simulink model "LongLatDriveline"  (R2024b)
settings: Solver=FixedStepAuto  StartTime=0  StopTime=120  FixedStep=0.002  RelTol=1e-3
InitFcn:
  | load('waypoints.mat');
  | VehicleObj = Simulink.data.dictionary.open('./ModelData/VehicleData.sldd');
  | %dDataSectObj = getSection(myDictionaryObj,'Design Data');
StopFcn:
  | Plot_LateralModelErrorControl;
  | 
  | mdlWks = get_param(gcs, 'ModelWorkspace');
  | par_ToDrvDesigner = evalin(mdlWks, 'ToDrvDesigner');
  | 
  | if par_ToDrvDesigner.Value
  |     ExportdrivingScenario;
  | end
model workspace (MAT data in the model file):
  ToDrvDesigner : Simulink.Parameter (value not decoded)
values from neighbouring files (symbols this model uses):
  A_F = 2.341157    [VehicleData.sldd]
  C_af = 80000.0    [VehicleData.sldd]
  C_ar = 80000.0    [VehicleData.sldd]
  C_d = 0.24    [VehicleData.sldd]
  f = 0.01    [VehicleData.sldd]
  g = 9.81    [VehicleData.sldd]
  h_aero = 0.65    [VehicleData.sldd]
  h_gc = 0.65    [VehicleData.sldd]
  Iz = 2873.0    [VehicleData.sldd]
  lf = 1.1    [VehicleData.sldd]
  lr = 1.58    [VehicleData.sldd]
  m = 2238.932    [VehicleData.sldd]
  Nf = 2.0    [VehicleData.sldd]
  Nr = 2.0    [VehicleData.sldd]
  r_stat = 0.342    [VehicleData.sldd]
  r_w = 0.352    [VehicleData.sldd]
  rho = 1.225    [VehicleData.sldd]
  theta = 0.0    [VehicleData.sldd]
  transGear = 0.1027    [VehicleData.sldd]
  V_wind = 0.0    [VehicleData.sldd]
symbols that are objects in the model workspace (value not decoded): ToDrvDesigner
undefined symbols (not defined in the file or in its folder): InitialPsi, InitialX, InitialY, phi
libraries: slpidlib x14, spsMosfetLib x6, simulink x4, spsVoltageMeasurementLib x3, SignalEditorBlockLib x2, spsDCVoltageSourceLib x1, spspowerguiLib x1
(part 3 of 5)

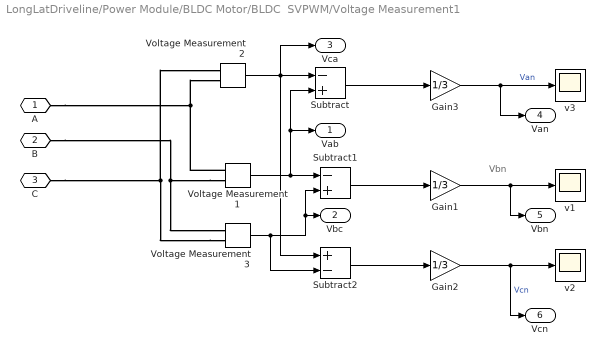
== system LongLatDriveline/Power Module/BLDC Motor/BLDC  SVPWM/Voltage Measurement1 ==
  note: Vbn
  Gain1 : Gain  Gain=1/3
  Gain2 : Gain  Gain=1/3
  Gain3 : Gain  Gain=1/3
  Subtract : Sum  Inputs=-+
  Subtract1 : Sum  Inputs=-+
  Subtract2 : Sum  Inputs=+-
  Voltage Measurement1 : spsVoltageMeasurementLib/Voltage Measurement  PhasorSimulation=off  OutputType=Complex  PSBequivalent=0
  Voltage Measurement2 : spsVoltageMeasurementLib/Voltage Measurement  PhasorSimulation=off  OutputType=Complex  PSBequivalent=0
  Voltage Measurement3 : spsVoltageMeasurementLib/Voltage Measurement  PhasorSimulation=off  OutputType=Complex  PSBequivalent=0
  v1 : Scope
  v2 : Scope
  v3 : Scope
  A : PMIOPort  Side=Left
  B : PMIOPort  Port=2  Side=Left
  C : PMIOPort  Port=3  Side=Left
  Vab : Outport  VectorParamsAs1DForOutWhenUnconnected=off
  Vbc : Outport  Port=2  VectorParamsAs1DForOutWhenUnconnected=off
  Vca : Outport  Port=3  VectorParamsAs1DForOutWhenUnconnected=off
  Van : Outport  Port=4  VectorParamsAs1DForOutWhenUnconnected=off
  Vbn : Outport  Port=5  VectorParamsAs1DForOutWhenUnconnected=off
  Vcn : Outport  Port=6  VectorParamsAs1DForOutWhenUnconnected=off
  wires:
  Gain2/1 -> v2/1, Vcn/1  "Vcn"
  Subtract2/1 -> Gain2/1
  Gain1/1 -> v1/1, Vbn/1
  Subtract1/1 -> Gain1/1
  Voltage Measurement3/1 -> Subtract1/2, Vbc/1, Subtract2/2
  Gain3/1 -> v3/1, Van/1  "Van"
  Subtract/1 -> Gain3/1
  Voltage Measurement1/1 -> Vab/1, Subtract/2, Subtract1/1
  Voltage Measurement2/1 -> Vca/1, Subtract2/1, Subtract/1
  connections:
  Voltage Measurement1/LConn1 -- A/RConn1 -- Voltage Measurement2/LConn2
  Voltage Measurement1/LConn2 -- B/RConn1 -- Voltage Measurement3/LConn1
  Voltage Measurement3/LConn2 -- Voltage Measurement2/LConn1 -- C/RConn1

== system LongLatDriveline/Vehicle Lateral Model/DynamicModel/LateralDynamics/LateralDynamicWithNoise ==
  note: This variant does not simplify the small angle tan. i.e. tan(x) = x
  X : Inport
  Vx : Inport  Port=2
  dd : Inport  Port=3
  phi_ref : Inport  Port=4
  LateralDynamicWithNoise : MATLAB Function  TreatAsAtomicUnit=on  VariantControl=NotSimplifiedModel
  Sine Wave : Sin  Amplitude=0.6  Frequency=(2*pi)/8  SampleTime=0
  Sine Wave1 : Sin  Amplitude=pi/60  Frequency=pi/8  SampleTime=0
  dX : Outport
  wires:
  X/1 -> LateralDynamicWithNoise/1(X)
  Vx/1 -> LateralDynamicWithNoise/2(Vx)
  dd/1 -> LateralDynamicWithNoise/3(dd)
  LateralDynamicWithNoise/1(dX) -> dX/1
  phi_ref/1 -> LateralDynamicWithNoise/4(phi_ref)
  Sine Wave/1 -> LateralDynamicWithNoise/5(NoiseDdy)
  Sine Wave1/1 -> LateralDynamicWithNoise/6(NoiseDdpsi)

== system LongLatDriveline/Power Module/BLDC Motor/BLDC  SVPWM/SVPWM Generator/Timer ==
  note: It triggers the output when the time is greatter or equal to the input in seconds
  time : Inport
  Add2 : Sum
  Constant13 : Constant
  Constant14 : Constant  Value=0
  Relational Operator : RelationalOperator  OutDataTypeStr=boolean  RndMeth=Simplest  InputSameDT=off
  Switch : Switch  Criteria=u2 > Threshold  SaturateOnIntegerOverflow=off  InputSameDT=off
  Unit Delay : UnitDelay  SampleTime=-1  HasFrameUpgradeWarning=on
  Weighted Sample Time : SampleTimeMath  TsampMathOp=Ts Only
  trigger : Outport
  wires:
  Switch/1 -> Unit Delay/1
  Add2/1 -> Relational Operator/1, Switch/3
  Relational Operator/1 -> trigger/1, Switch/2
  Weighted Sample Time/1 -> Add2/1
  Constant13/1 -> Weighted Sample Time/1
  Constant14/1 -> Switch/1
  Unit Delay/1 -> Add2/2
  time/1 -> Relational Operator/2

== system LongLatDriveline/Power Module/BLDC Motor/BLDC  SVPWM/SVPWM Generator/count14 ==
  Trigger : TriggerPort  VariantControl=(inherit)
  Add : Sum
  Compare To Constant : simulink/Logic and Bit Operations/Compare To Constant  relop=>=  const=4  OutDataTypeStr=boolean
  Compare To Constant1 : simulink/Logic and Bit Operations/Compare To Constant  relop=<=  const=1  OutDataTypeStr=boolean
  Constant : Constant  Value=-1
  Constant1 : Constant
  Switch : Switch  Criteria=u2 > Threshold  Threshold=1  SaturateOnIntegerOverflow=off  InputSameDT=off
  Switch1 : Switch  Criteria=u2 > Threshold  Threshold=1  SaturateOnIntegerOverflow=off  InputSameDT=off
  Unit Delay : UnitDelay  InitialCondition=1  SampleTime=-1  HasFrameUpgradeWarning=on
  Unit Delay1 : UnitDelay  InitialCondition=1  SampleTime=-1  HasFrameUpgradeWarning=on
  count : Outport  InitialOutput=1
  wires:
  Add/1 -> Unit Delay/1, count/1, Compare To Constant/1, Compare To Constant1/1
  Unit Delay/1 -> Add/2
  Unit Delay1/1 -> Switch/3, Add/1
  Constant/1 -> Switch/1
  Switch/1 -> Switch1/3
  Switch1/1 -> Unit Delay1/1
  Compare To Constant/1 -> Switch/2
  Compare To Constant1/1 -> Switch1/2
  Constant1/1 -> Switch1/1

== matlab function LongLatDriveline/Tyre ModelV1/TireSlip ==
  data: Vx input; s_xf output; w_wf input; r_eff input
%BASED ON
%Rajesh Rajamani, Vehicle Dynamics and Control, Minneapolis, MN, Springer, 2012.
%Chapter 4.1.2
function s_xf = XTireSlip(Vx,w_wf,r_eff) 

if Vx == 0
   s_xf = 0.1 * sign(w_wf);   
else
   s_xf = (r_eff*w_wf -Vx)/abs(Vx); % acceleration
end

if s_xf > 1
   %s_xf = 1; 
end

== matlab function LongLatDriveline/LateralController/SMC_Alcala/AlcalaSMC ==
  data: U output size=1; E input; Vx input; dPsi_des input; dx_e input; ddPsi_des input; C_af parameter; g parameter; C_ar parameter; lf parameter; lr parameter; Iz parameter; m parameter
% ******************* Lateral dynamic controller *********************
%*********************************************************************
% Author: L.Arturo Torres-Romero
% Date: 22-10-2020
% This controller controlls the direction of a car, based in the dynamics
% described  in the next link and using the Direct Lyapunov formulation: 
% https://www.researchgate.net/publication/340166902_LATERAL_VEHICLE_DYNAMICS_AND_CONTROLLERS_DESIGN
%
%ALCALÁ, Eugenio, et al. Comparison of two non-linear model-based control strategies for autonomous vehicles. 
% En 2016 24th Mediterranean Conference on Control and Automation (MED). IEEE, 2016. p. 846-851.
%******************* PARAMETERS DESCRIPTIONS **********************
%******************************************************************
% m: vehicle mass
% g: gravity
% C_af : Cornering  stiffness  of  front  wheels.
% C_ar : Cornering  stiffness  of  rear  wheels.
% lf : distance fron the center of gravity to the front wheel axis.
% lr : distance fron the center of gravity to the rear wheel axis.
% Iz : this is the momentum of inertia of the vehicle respect the z axis.
%******************************************************************
%******************* INPUTS DESCRIPTIONS **************************
%******************************************************************
% E:   (column vector)[e1;de1;e2;de2] states of the state space of 
%       the system that includes the errors as follows:
%      e1  : is the lateral position error respect the road.
%      de1 : derivative of e1.
%      e2  : is the yaw angle error with respect the road. 
%      de2 : derivarive of the e2.
% Vx: Logitudinal velocity.

%******************************************************************
% ******************* OUTPUTS DESCRIPTIONS ************************
%******************************************************************
% U: control coutput in radians. Angle of the frontal wheels respect to the
%    longitudinal axis
% isCtrl: when true means that the matrix Mc has full rank, and hence, the
%         system is controllable
%******************************************************************

function U = SMC_Ctrl_1(E, Vx,dPsi_des,dx_e,ddPsi_des, C_af, g, C_ar, lf, lr, Iz, m) % pd polos deseados
y_e = E(1);
dy_e = E(2);
psi_e = E(3);
dpsi_e = E(4);
x_e = E(5);


L = lf+lr;
k2 = 2;
k3 = 2.55;
P2 = 3.7;
Q2 = 0.3;

s2 = dy_e +k2*y_e + k3*psi_e;

dPsi_ctrl = dPsi_des + (-P2*s2 -Q2*sign(s2) -k2*dy_e + ddPsi_des*x_e + dPsi_des*dx_e  -Vx*sin(psi_e))/(Vx*sin(psi_e)+k3);

ctrlVal = atan((L*dPsi_ctrl)/Vx);

U = real(ctrlVal);

== matlab function LongLatDriveline/Tyre ModelV1/WheelsDynamic ==
  data: T_wheels input; dw_wf output; r_eff output; F_xf input; r_w parameter; r_stat parameter
% ******************* Wheel inertia dynamics *********************
%****************************************************************
% BASED ON 
% Rajesh Rajamani, Vehicle Dynamics and Control, Minneapolis, MN, Springer, 2012.
%Chapter 4.2.4
% r_eff = effective radius of the wheel
% F_xf = longitudinal tire force from the front wheels
function [dw_wf, r_eff]= fcn(T_wheels,F_xf, r_w, r_stat)

%r_w = 0.352; % radius of the tire. Pirelli Sottozero 3 P245/45WR19
%r_stat = 0.342; % static vertical deflection of the tire
alpha = acos(r_stat/r_w);
r_eff = (alpha*r_w)/alpha;

I_w = .9; % TODO define this
dw_wf = (T_wheels -(r_eff*F_xf))/I_w;

== matlab function LongLatDriveline/Power Module/BLDC Motor/BLDC  SVPWM/InvPark ==
  data: X_dq input size=[2 1]; Y_ab0 output; theta input
function Y_ab0 = fcn(X_dq, theta)
X_dq0 = [X_dq; 0];

%inverse Park 
iT_C = [cos(theta)   -sin(theta)    0; ...
        sin(theta)    cos(theta)    0; ...
        0             0             1];
%               
             
Y_ab0 =iT_C*X_dq0;
end

== matlab function LongLatDriveline/Tyre ModelV2/MagicFormula ==
  data: X input; Y output; F_zf input
%BASED ON
%Massimo Guiggiani, The Science of Vehicle Dynamics, Pisa, Italy, Springer Netherlands, 2014.
%Chapter 2.12
%The values of the MF were obtained from the graph in fig. 2.22
function Y = XTireForce(X, F_zf) 
% B stiffness factor
% C shape factor
% D peak value
% E curvature factor
% Sh horizontal shift
% Sv vertical shift

Sh = 0;% Sh horizontal shift
Sv = 0; %vertical shift

D = 3; % ym, maximum value Experimental from graph
C = 1.5;
B = 20;
E = 0;

x = X-Sh;
gamma = C*atan(B*x-E*(B*x-atan(B*x)));
y = F_zf*D*sin(gamma);
Y = (y - Sv);

== matlab function LongLatDriveline/Tyre ModelV2/TireSlip ==
  data: Vx input; s_xf output; w_wf input; r_eff input
%BASED ON
%Rajesh Rajamani, Vehicle Dynamics and Control, Minneapolis, MN, Springer, 2012.
%Chapter 4.1.2
function s_xf = XTireSlip(Vx,w_wf,r_eff) 

if Vx == 0
   s_xf = 0.1 * sign(w_wf);   
else
   s_xf = (r_eff*w_wf -Vx)/abs(Vx); % acceleration
end

if s_xf > 1
   %s_xf = 1; 
end

== matlab function LongLatDriveline/Power Module/SIEngineModel/SI_Engine/FrictionLosses ==
  data: w_e input; T_f output; p_man input
function T_f = fcn(w_e, p_man)
% According Heywood 98 friction loss = .97 +0.15*(N/1000)+  0.05(N/1000)^2
% Where N is RPM. here it is converted to rad/s



a0 = 4.559432e-6;
a1 = 0.009550;
a2 = .97;
b0 = 0;
b1 = 0;




T_f = abs(a0*w_e^2 + a1*w_e + a2 + b0*w_e*p_man + b1*p_man);a1*w_e + a2 + b0*w_e*p_man + b1*p_man;

== matlab function LongLatDriveline/Power Module/BLDC Motor/BLDC  SVPWM/MATLAB Function ==
  data: r output; x input; theta output; y input
function [r, theta] = rec2polar(x, y)

r = sqrt(x^2 + y^2);
theta = atan2(y,x);

== matlab function LongLatDriveline/Power Module/DC Motor/DC Motor ==
  data: X input; dX output; u input size=3; T output
function [dX, T]= fcn(X,u)
ia = X(1);
Va = u(1); wm =u(2); dwm =u(3);

MaxT = 800;

Ra = 0.193;
La = 0.00383;
Jm = 0.6;
Bm = 2.632177;
Kb = 2.332232;
KT = 2.1717;

A1 = -Ra/La;
B1 = [1/La -Kb/La 0];
C1 = KT;
D1 = [0 -Bm -Jm];

dX = A1*X + B1*u;
T = C1*X + D1*u;

if T > MaxT
    T = MaxT;
end
if T < 0
    T = 0;
end

end

== matlab function LongLatDriveline/Power Module/SIEngineModel/SI_Engine/InflowRateManifold ==
  data: alpha input; dm_ai output; p_man input
function dm_ai = fcn(alpha,p_man)

% Max  Automotive Powertrain Modeling for Control (D.Cho and J. K. Hedrick)
MAX = 0.1843; % Kg/s constant dependent on the size of the throttle body and is equalto the maximum possible intake airflow rate.
alpha_p = 0.05; %the minimum throttle angle seen by the engine.
pc = 0.5283; % critical pressure ratio
p_amb =101325; % pressure of 1 atm in Pa
p_r = p_man/p_amb;

if p_r <= pc
PRI = 1; % p_r <= pc Sonic
else
PRI = sqrt(1-((p_r-pc)/(1-pc))^2); % P_r > pc   chocked
end

TC = 1-cos(alpha-alpha_p);
dm_ai = MAX * TC * PRI;

== matlab function LongLatDriveline/Power Module/SIEngineModel/SI_Engine/ManifoldPressure ==
  data: dm_ao input; dm_ai input; dp_man output
function dp_man = fcn(dm_ao,dm_ai)
R = 8.314472; % (J/(K*mol)) ideal gas constant.
T_man = 60; % intake manifold temperature.
V_man = 1; % intake manifold volume

dp_man = (R*T_man*(dm_ai-dm_ao))/V_man;

== matlab function LongLatDriveline/LongitudinalDynamics ==
  data: F_xf input; dVx output; F_xr input; Vx input; rho parameter; g parameter; A_F parameter; C_d parameter; f parameter; m parameter; V_wind parameter; theta parameter; F_zf output; F_zr output; h_aero parameter; h_gc parameter; lf parameter; lr parameter; Nf parameter; Nr parameter
% BASED ON
% Rajesh Rajamani, Vehicle Dynamics and Control, Minneapolis, MN, Springer, 2012.
%Chapter 4.1

function [dVx,F_zf, F_zr] = LongitudinalDynamics(F_xf,F_xr,Vx, rho, g, A_F, C_d, f, m, V_wind, theta, h_aero, h_gc, lf, lr, Nf, Nr)
% m = 2238.932; % TESLA model S P85D
% g = 9.81;
% theta = 0;
% A_F = 2.341157; % Fontal area of the vehicle. TESLA model S P85D
% C_d  =0.24; %Ford Focus Aerodynamic drag coeficient. TESLA model S P85D
% rho = 1.225;  %(kg/m^3) Air density
% f = 0.01; % varies from 0.01 to 0.04
% V_wind = 0;
% Nf, Nr Number of wheels in front and rear axles

F_aero = (1/2)*rho*C_d*A_F*(Vx+V_wind)^2;

dVx = (F_xf + F_xr - F_aero - m*g*sin(theta))/m;

F_zf = (-F_aero*h_aero -m*dVx*h_gc -m*g*h_gc*sin(theta) +m*g*lr*cos(theta))/(Nf*(lr+lf));
F_zr = ( F_aero*h_aero +m*dVx*h_gc +m*g*h_gc*sin(theta) +m*g*lf*cos(theta))/(Nr*(lr+lf));

== matlab function LongLatDriveline/Power Module/SIEngineModel/SI_Engine/OutflowRateManifold ==
  data: w_e input; dm_ao output; p_man input; T_man input; ma input
function dm_ao = fcn(w_e, p_man, T_man,ma)
Vd = 0.0038; %displacement volume of the engine cylinders
R = 8.31446261815324; %constant used in ideal gas law for intake manifold

%volumetric efficiency

% Automotive Powertrain Modeling for Control (D.Cho and J. K. Hedrick)
eta_vol = (24.5*w_e -3.1e4)*ma^2 + (-1.167*w_e+222)*ma +(8.1e-4*w_e+0.352);
%eta_vol = 0.9;

dm_ao = ((eta_vol*w_e*Vd)/(4*pi))*(p_man/(R*T_man));

== matlab function LongLatDriveline/Power Module/SIEngineModel/SI_Engine/indTorque ==
  data: w_e input; T_ind output; dm_ao input
function T_ind = fcn(w_e, dm_ao)
% dm_ao: air mass flow rate out of the intake manifold and into the cylinder
% dm_f:  is the mass fuel rate into the cylinders 
H_u = 46000000; % fuel energy constant. look in other sources 44-46 MJ/kg found as (Gasoline heating value)
h_i = 0.45; % Thermal efficiency multiplier. Otto engine value.   from (Hendricks and Sorenson, 1990)
lambda = 1; % air/fuel equivalence ratio
L_th = 14.67; % stoichiometric air/fuel mass ratio for gasoline.


dm_f = dm_ao/(L_th*lambda);

if w_e ~= 0
T_ind = (H_u*h_i*dm_f)/w_e;   
else
T_ind = (H_u*h_i*dm_f)/0.01;    
end

== matlab function LongLatDriveline/Power Module/BLDC Motor/BLDC  SVPWM/Motor BLDC1 ==
  data: X input; dX output; Fabc input; u input; Wm input; dWm input; Tl output
function [dX, Tl] = fcn(X, Fabc, u, Wm, dWm)

== matlab function LongLatDriveline/Tyre ModelV2/WheelsDynamic ==
  data: T_wheels input; dw_wf output; r_eff output; F_xf input; r_w parameter; r_stat parameter
% ******************* Wheel inertia dynamics *********************
%****************************************************************
% BASED ON 
% Rajesh Rajamani, Vehicle Dynamics and Control, Minneapolis, MN, Springer, 2012.
%Chapter 4.2.4
% r_eff = effective radius of the wheel
% F_xf = longitudinal tire force from the front wheels
function [dw_wf, r_eff]= fcn(T_wheels,F_xf, r_w, r_stat)

%r_w = 0.352; % radius of the tire. Pirelli Sottozero 3 P245/45WR19
%r_stat = 0.342; % static vertical deflection of the tire
alpha = acos(r_stat/r_w);
r_eff = (alpha*r_w)/alpha;

I_w = .9; % TODO define this
dw_wf = (T_wheels -(r_eff*F_xf))/I_w;

== matlab function LongLatDriveline/Power Module/BLDC Motor/BLDC  SVPWM/ParkClarke4 ==
  data: X_abc input; Y_dq output; theta input
function Y_dq = fcn(X_abc, theta)

% Park clarke transform eliminating the third element
PC_T = (sqrt(2)/2)*[sqrt(3)*cos(theta)  sin(theta)  -sin(theta) ; ...
                    -sqrt(3)*sin(theta)  cos(theta)  -cos(theta)];

Y_dq =PC_T*X_abc;
end

== matlab function LongLatDriveline/Power Module/BLDC Motor/BLDC  SVPWM/SVPWM Generator/bin2vector ==
  data: y output; data input
function y = binary2vector(data)
y = [0; 0; 0];
g = dec2bin(data,3);
out = g-'0';
y(1) = out(1);
y(2) = out(2);
y(3) = out(3);


% powOf2 = 2.^[0:nBits-1];
% 
% %# do a tiny bit of error-checking
% if data > sum(powOf2)
%    error('not enough bits to represent the data')
% end
% 
% out = false(1,nBits);
% 
% ct = nBits;
% 
% while data>0
% if data >= powOf2(ct)
% data = data-powOf2(ct);
% out(ct) = true;
% end
% ct = ct - 1;
% end

== matlab function LongLatDriveline/Power Module/BLDC Motor/BLDC  SVPWM/Space Vector calculator ==
  data: n output; v output; theta_vs output; V_link input; Vs input; theta_vs1 input
function [n,v,theta_vs]= SpaceVectorCalc(V_link,Vs,theta_vs1)
v = [0 0];
theta_vs = mod(theta_vs1,2*pi);
theta = 0;
n = 0; % This is the quadrant of the vector. you should never get zero as output

if 0*(pi/180) <= theta_vs && theta_vs < 60*(pi/180)
   theta = theta_vs;
   n = 1;
elseif 60*(pi/180) <= theta_vs && theta_vs < 120*(pi/180)
   theta = theta_vs - 60*(pi/180);
   n = 2;
elseif 120*(pi/180) <= theta_vs && theta_vs < 180*(pi/180)  
    theta = theta_vs - 2*60*(pi/180);
    n = 3;
elseif 180*(pi/180) <= theta_vs && theta_vs < 240*(pi/180)  
    theta = theta_vs - 3*60*(pi/180);
    n = 4;
elseif 240*(pi/180) <= theta_vs && theta_vs < 300*(pi/180)
    theta = theta_vs - 4*60*(pi/180);
    n = 5;
elseif 300*(pi/180) <= theta_vs && theta_vs < 360*(pi/180)
    theta = theta_vs - 5*60*(pi/180);
    n = 6;
end


V_b = ((2*Vs)/sqrt(3))*sin(theta);
V_a = ((2*Vs)/sqrt(3))*sin(pi/3 - theta);

v = [V_a V_b];

== matlab function LongLatDriveline/Transmission ==
  data: T_wheels output; T_t input; w_t output; w_w input; R input
% ***************** Transmission ******************
% *************************************************
% BASED ON
% Rajesh Rajamani, Vehicle Dynamics and Control, Minneapolis, MN, Springer, 2012.
% Chapter 4.2.2
% T_wheels = wheels torque
% w_w = wheels angular speed
% R = gear ratio of transmission
%**************************************************

function [T_wheels, w_t]= fcn(T_t,w_w,R)

T_wheels = T_t/R;
w_t = w_w/R;
% itneed to be implemented "during change"

== matlab function LongLatDriveline/Power Module/BLDC Motor/BLDC abcModel/Fases abc ==
  data: X input; Fabc output
function Fabc = fcn(X)
    theta = mod(X(1),2*pi);
    
    if (0<=theta)&&(theta<(pi/6))
        Fa = (6/pi)*theta;
    elseif ((pi/6)<=theta)&&(theta<(5*pi/6))
        Fa = 1;
    elseif ((5*pi/6<=theta))&&(theta<(7*pi/6))
        Fa = (6/pi)*(pi-theta);
    elseif ((7*pi/6)<=theta)&&(theta<(11*pi/6))
        Fa = -1;
    elseif ((11*pi/6)<=theta)&&(theta<(2*pi))
        Fa = (6/pi)*(theta-2*pi);
    else
        Fa = NaN;
    end
    
    if (0<=theta)&&(theta<(3*pi/6))
        Fb = -1;
    elseif ((3*pi/6)<=theta)&&(theta<(5*pi/6))
        Fb = (6/pi)*(theta-(2*pi)/3);
    elseif ((5*pi/6)<=theta)&&(theta<(9*pi/6))
        Fb = 1;
    elseif ((9*pi/6)<=theta)&&(theta<(11*pi/6))
        Fb = (6/pi)*(-theta+(5*pi)/3);
    elseif ((11*pi/6)<=theta)&&(theta<(2*pi))
        Fb = -1;
    else
        Fb = NaN;
    end
    
    if (0<=theta)&&(theta<(pi/6))
        Fc = 1;
    elseif ((pi/6)<=theta)&&(theta<(3*pi/6))
        Fc = (6/pi)*(pi/3-theta);
    elseif ((3*pi/6)<=theta)&&(theta<(7*pi/6))
        Fc = -1;
    elseif ((7*pi/6)<=theta)&&(theta<(9*pi/6))
        Fc = (6/pi)*(theta-(4*pi)/3);
    elseif ((9*pi/6)<=theta)&&(theta<(2*pi))
        Fc = 1;
    else
        Fc = NaN; 
    end
    
    Fabc = [Fa;Fb;Fc];
end

== matlab function LongLatDriveline/Power Module/BLDC Motor/BLDC abcModel/Graphs ==
  data: X input; theta output; Iabc output
function [theta,Iabc] = DEMUX(X)
theta = X(1);Iabc = X(2:4);

== matlab function LongLatDriveline/Power Module/BLDC Motor/BLDC abcModel/Motor BLDC ==
  data: X input; dX output; Fabc input; u input; Wm input; dWm input; Tl output
function [dX,Tl] = fcn(X,Fabc,u,Wm,dWm)
Iabc = X(2:4);
R = 0.7;
L = 0.005;%0.00272-0.0015; %=L-Lm
J = 0.000284;
b = 0.02;
P = 4;
maxTl = 400; % max torque of the motor
Lambda = 0.105;

Vabc = u*Fabc;

Eabc = Lambda*Wm*Fabc;
dTheta = P*Wm/2;

if Wm > 0.01
Te = (Iabc'*Eabc)/Wm;
Tl = Te-b*Wm-J*dWm;
else
Tl  = maxTl;
end

if Tl > maxTl
Tl = maxTl;   
end

dIabc = (-R*Iabc - Eabc + Vabc)/L;

dX = [dTheta;dIabc];
end

== matlab function LongLatDriveline/Power Module/BLDC Motor/BLDC dqControl/Back EMF ==
  data: X input; Fabc output
function Fabc = fcn(X)
Fabc = [0;0;0];
    theta = mod(X(1),2*pi); %X(4)
    %theta = mod(X,2*pi);
    
    if (0<=theta)&&(theta<(pi/6))
        Fa = (6/pi)*theta;
    elseif ((pi/6)<=theta)&&(theta<(5*pi/6))
        Fa = 1;
    elseif ((5*pi/6<=theta))&&(theta<(7*pi/6))
        Fa = (6/pi)*(pi-theta);
    elseif ((7*pi/6)<=theta)&&(theta<(11*pi/6))
        Fa = -1;
    elseif ((11*pi/6)<=theta)&&(theta<(2*pi))
        Fa = (6/pi)*(theta-2*pi);
    else
        Fa = NaN;
    end
    
    if (0<=theta)&&(theta<(3*pi/6))
        Fb = -1;
    elseif ((3*pi/6)<=theta)&&(theta<(5*pi/6))
        Fb = (6/pi)*(theta-(2*pi)/3);
    elseif ((5*pi/6)<=theta)&&(theta<(9*pi/6))
        Fb = 1;
    elseif ((9*pi/6)<=theta)&&(theta<(11*pi/6))
        Fb = (6/pi)*(-theta+(5*pi)/3);
    elseif ((11*pi/6)<=theta)&&(theta<(2*pi))
        Fb = -1;
    else
        Fb = NaN;
    end
    
    if (0<=theta)&&(theta<(pi/6))
        Fc = 1;
    elseif ((pi/6)<=theta)&&(theta<(3*pi/6))
        Fc = (6/pi)*(pi/3-theta);
    elseif ((3*pi/6)<=theta)&&(theta<(7*pi/6))
        Fc = -1;
    elseif ((7*pi/6)<=theta)&&(theta<(9*pi/6))
        Fc = (6/pi)*(theta-(4*pi)/3);
    elseif ((9*pi/6)<=theta)&&(theta<(2*pi))
        Fc = 1;
    else
        Fc = NaN; 
    end
    
    
%     
     %Fa = sin(theta);
     %Fb = sin(theta - 2*pi/3);
     %Fc = sin(theta + 2*pi/3);
    
    Fabc = [Fa;Fb;Fc];
end

== matlab function LongLatDriveline/LateralController/SMC_UrbanoPathFollowing/SMC_UrbanoPathFollowing ==
  data: U output size=1; E input; Vx input; dPsi_des input; d_d input; C_af parameter; g parameter; C_ar parameter; lf parameter; lr parameter; Iz parameter; m parameter; dd_d output
% ******************* Lateral dynamic controller *********************
%*********************************************************************
% Author: L.Arturo Torres-Romero
% Date: 22-10-2023
% This controller controlls the direction of a car, based on the path
% following controller described  in the next paper and link: 
%
%SOLEA, Razvan; NUNES, Urbano. Trajectory planning and sliding-mode control based trajectory-tracking for cybercars. 
% Integrated Computer-Aided Engineering, 2007, vol. 14, no 1, p. 33-47.
%
%https://www.researchgate.net/publication/228634486_Trajectory_planning_and_sliding-mode_control_based_trajectory-tracking_for_cybercars
%SOLEA, Razvan; NUNES, Urbano. Trajectory planning and sliding-mode control based trajectory-tracking for cybercars.
%Integrated Computer-Aided Engineering, 2007, vol. 14, no 1, p. 33-47.
%
%******************* PARAMETERS DESCRIPTIONS **********************
%******************************************************************
% m: vehicle mass
% g: gravity
% C_af : Cornering  stiffness  of  front  wheels.
% C_ar : Cornering  stiffness  of  rear  wheels.
% lf : distance fron the center of gravity to the front wheel axis.
% lr : distance fron the center of gravity to the rear wheel axis.
% Iz : this is the momentum of inertia of the vehicle respect the z axis.
%******************************************************************
%******************* INPUTS DESCRIPTIONS **************************
%******************************************************************
% E:   (column vector)[e1;de1;e2;de2] states of the state space of 
%       the system that includes the errors as follows:
%      e1  : is the lateral position error respect the road.
%      de1 : derivative of e1.
%      e2  : is the yaw angle error with respect the road. 
%      de2 : derivarive of the e2.
% Vx: Logitudinal velocity.

%******************************************************************
% ******************* OUTPUTS DESCRIPTIONS ************************
%******************************************************************
% U: control coutput in radians. Angle of the frontal wheels respect to the
%    longitudinal axis
%******************************************************************

function [U, dd_d] = SMC_Ctrl_1(E, Vx,dPsi_des, d_d, C_af, g, C_ar, lf, lr, Iz, m) % pd polos deseados
y_e = E(1);
dy_e = E(2);
psi_e = E(3);
dpsi_e = E(4);

L = lf+lr;
k = 0.5;
k0 = 0.05;
q1 = 1;
q2 = 1;
p1 = 1;
p2 = 1;
Lh = 6.5; % this lenght was obtained based in the 5 points ahead of the C.G. for refference aprx. See GetRefference block

s = dy_e + k*y_e + k0*sign(y_e)*psi_e;

if Lh == 0   % Look-ahead = 0. TODO
    ctrlVal = 0;


else   % Look-ahead <> 0|
    Q = q1;
    P = p1;
    tmp1 = (L*(cos(d_d))^2)/(Vx*Lh*cos(dpsi_e)^2);
    tmp2 = -Q*s -P*sign(s)-k*dy_e -Vx*dpsi_e*cos(psi_e) + Lh*dpsi_e^2*sin(psi_e) - k0*sign(y_e)*dpsi_e;
    dd_d = tmp1*tmp2;
    ctrlVal = real(d_d); 
end

U = real(ctrlVal);

== matlab function LongLatDriveline/Power Module/BLDC Motor/BLDC dqControl/InvParkClarke ==
  data: X_dq input; Y_abc output; theta input
function Y_abc = fcn(X_dq, theta)
X_dq0 = [X_dq; 0];

%inverse Park-Clarke power invariant
iT_PC = sqrt(2/3)*[cos(theta)          -sin(theta)            1/sqrt(2); ...
                  cos(theta-2*pi/3)   -sin(theta-2*pi/3)     1/sqrt(2); ...
                  cos(theta+2*pi/3)   -sin(theta+2*pi/3)     1/sqrt(2)];
%               
              
 %inverse Park-Clarke amplitude invariant
% iT_PC = [cos(theta)          -sin(theta)            1; ...
%          cos(theta-2*pi/3)   -sin(theta-2*pi/3)     1; ...
%          cos(theta+2*pi/3)   -sin(theta+2*pi/3)     1];


Y_abc = [0;0;0];
Y_abc =iT_PC*X_dq0;
end

== matlab function LongLatDriveline/Power Module/BLDC Motor/BLDC dqControl/Motor BLDC1 ==
  data: X input; dX output; Fabc input; u input; Wm input; dWm input; Tl output
function [dX,Tl] = fcn(X,Fabc,u,Wm,dWm)
Iabc = X(2:4);
R = 0.0075;% ohms
L = 0.00183;% H      0.00272-0.0015; %=L-Lm
J = 0.04; % kg/m^2
b = 0.27285; %0.02; Nm
P = 4; % poles
maxTl = 430; % max torque of the motor
Lambda = 0.0836;

Vabc = u;

Eabc = Lambda*Wm*Fabc;
dTheta = P*Wm/2;

if Wm > 0.01
Te = (Iabc'*Eabc)/Wm;
Tl = Te-b*Wm-J*dWm;
else
Tl  = maxTl;
end

if abs(Tl) > maxTl
Tl = maxTl*sign(Tl);   
end

dIabc = (-R*Iabc - Eabc + Vabc)/L;

dX = [dTheta;dIabc];
end

== matlab function LongLatDriveline/Power Module/BLDC Motor/BLDC dqControl/ParkClarke ==
  data: X_abc input; Y_dq output; theta input
function Y_dq = fcn(X_abc, theta)

% Park clarke transform eliminating the third element
PC_T = (sqrt(2)/2)*[sqrt(3)*cos(theta)  sin(theta)  -sin(theta) ; ...
                    -sqrt(3)*sin(theta)  cos(theta)  -cos(theta)];

Y_dq =PC_T*X_abc;
end

== matlab function LongLatDriveline/MATLAB Function ==
  data: u input; y output
function y = ms2kmh(u)

y = (u*60*60)/1000;

== matlab function LongLatDriveline/LateralController/AckermanCtrl ==
  data: U output size=1; E input; Vx input; C_af parameter; g parameter; C_ar parameter; lf parameter; lr parameter; Iz parameter; m parameter
% ******************* Lateral dynamic controller *********************
%*********************************************************************
% Author: L.Arturo Torres-Romero
% Date: 22-10-2020
% This controller controlls the direction of a car, based in the dynamics
% described  in the next link and using the Ackerman formulation: 
% https://www.researchgate.net/publication/340166902_LATERAL_VEHICLE_DYNAMICS_AND_CONTROLLERS_DESIGN
%******************* PARAMETERS DESCRIPTIONS **********************
%******************************************************************
% m: vehicle mass
% g: gravity
% C_af : Cornering  stiffness  of  front  wheels.
% C_ar : Cornering  stiffness  of  rear  wheels.
% lf : distance fron the center of gravity to the front wheel axis.
% lr : distance fron the center of gravity to the rear wheel axis.
% Iz : this is the momentum of inertia of the vehicle respect the z axis.
%******************************************************************
%******************* INPUTS DESCRIPTIONS **************************
%******************************************************************
% E:   (column vector)[e1;de1;e2;de2] states of the state space of 
%       the system that includes the errors as follows:
%      e1  : is the lateral position error respect the road.
%      de1 : derivative of e1.
%      e2  : is the yaw angle error with respect the road. 
%      de2 : derivarive of the e2.
% Vx: Logitudinal velocity.

%******************************************************************
% ******************* OUTPUTS DESCRIPTIONS ************************
%******************************************************************
% U: control coutput in radians. Angle of the frontal wheels respect to the
%    longitudinal axis
% isCtrl: when true means that the matrix Mc has full rank, and hence, the
%         system is controllable
%******************************************************************

function U = AckermanLateralCtrl(E, Vx, C_af, g, C_ar, lf, lr, Iz, m) % pd polos deseados
X = [0; 0; 0; 0];
X(1) = E(1);
X(2) = E(2);
X(3) = E(3);
X(4) = E(4);
%**************************************************
%******* Matrix A formulation *********************
A22 = -(2*C_af + 2*C_ar)/(m*Vx);
A23 = (2*C_af + 2*C_ar)/m;
A24 = (-2*C_af*lf + 2*C_ar*lr)/(m*Vx);
A42 = -(2*C_af*lf - 2*C_ar*lr)/(Iz*Vx);
A43 = (2*C_af*lf - 2*C_ar*lr)/Iz;
A44 = -(2*C_af*lf^2 + 2*C_ar*lr^2)/(Iz*Vx);

A = [0 1 0 0;0 A22 A23 A24;0 0 0 1;0 A42 A43 A44];
%**************************************************

%**************************************************
%******* Matrix B1 formulation ********************
B1_2 = 2*C_af/m;
B1_4 = 2*C_af*lf/Iz;

B1 = [0;B1_2;0;B1_4];
%***************************************************

%***************************************************
%******* Matrix B2 formulation *********************
B2_2 = -(2*C_af*lf - 2*C_ar*lr)/(m*Vx) - Vx;
B2_4 = -(2*C_af*lf^2 + 2*C_ar*lr^2)/(Iz*Vx);

B2 = [0;B2_2;0;B2_4];
%***************************************************


%***************************************************
%******* Matrix B3 formulation *********************
B3 = [0;g;0;0];
%***************************************************


%***************************************************
%******* Verification of controllability and output 
% calculation of the controller
%**************************************************
ctrlVal = 0;
Mc = [B1 A*B1 A^2*B1 A^3*B1];
rankVal = rank(Mc);
    if rankVal < size(A,1)
        %disp('Not completely state controllable');
        isCtrl = 0;
        ctrlVal = 0;
    else
        %disp('Completely state controllable');
        isCtrl = 1;
        % Pole placement
        Pd =[-10-3i -8+3i -15 -19]; %[-5-3i -5+3i -7 -10]
        %Pd =[-2 -2 -2 -2];

        H = (A- Pd(1)*eye(4)) * (A- Pd(2)*eye(4)) * (A- Pd(3)*eye(4)) * (A- Pd(4)*eye(4));

        %ackerman formula
        K = [0 0 0 1]*Mc^-1*H;
        ctrlVal = -K*X;  
    end


U = real(ctrlVal);

== matlab function LongLatDriveline/LateralController/SMC_Alcala/LevantDiff/Levant ==
  data: dX output; X input; u_ref input; lambda input; alpha input
%*************************************************
% Author: L.Arturo Torres-Romero
% based on 
% Levant A. (1998). Robust exact differentiation via sliding mode technique. 
% Automatica, 34(3), 379-384
%*************************************************

function dX = LevantDiff(X, u_ref, lambda, alpha) 
eta_u0=X(1);    eta_u1= X(2); 

 
%Levant differenciator
 d_eta_u0=eta_u1-lambda*sqrt(abs(eta_u0-u_ref))*sign(eta_u0-u_ref);
 d_eta_u1=-alpha*sign(eta_u0-u_ref);
      
dX = [d_eta_u0;d_eta_u1];
end

== matlab function LongLatDriveline/LateralController/SMC_Alcala/LevantDiff1/Levant ==
  data: dX output; X input; u_ref input; lambda input; alpha input
%*************************************************
% Author: L.Arturo Torres-Romero
% based on 
% Levant A. (1998). Robust exact differentiation via sliding mode technique. 
% Automatica, 34(3), 379-384
%*************************************************

function dX = LevantDiff(X, u_ref, lambda, alpha) 
eta_u0=X(1);    eta_u1= X(2); 

 
%Levant differenciator
 d_eta_u0=eta_u1-lambda*sqrt(abs(eta_u0-u_ref))*sign(eta_u0-u_ref);
 d_eta_u1=-alpha*sign(eta_u0-u_ref);
      
dX = [d_eta_u0;d_eta_u1];
end

== matlab function LongLatDriveline/SteerActuator/BLDCWRack/BLDC_AngleCtrl2/BLDC abc model ==
  data: X input; f input; v input; dX output; Tl input; R parameter; L parameter; M parameter; J parameter; b parameter; P parameter; lambda parameter
function dX = fcn(X,f,v,Tl, R, L, M, J, b, P, lambda)
% X = [i_a; i_b; i_c; wm; theta_elec]
% f = [f1; f2; f3]  (0..1)
% v = [v1; v2; v3]  (example v = 12.*f)
% Tl = scalar torque load)
% lambda = ke = kt (V·s/rad = N·m/A)
% P = poles qty (pole pairs = P/2
%
% delivers dX = [di_a; di_b; di_c; dwm; dtheta_elec]

% sanity checks
if numel(f)~=3 || numel(v)~=3
    error('f and v must be vectors 3x1.');
end

% effective electric parameters
L_eff = L - M;
if L_eff <= 0
    error('L - M must be possitive. Check M.');
end


% states
i_a = X(1); i_b = X(2); i_c = X(3);
wm  = X(4); theta = X(5);


% electric equations (phase to phase)
di_a = ( v(1) - R*i_a - lambda * f(1) * wm ) / L_eff;
di_b = ( v(2) - R*i_b - lambda * f(2) * wm ) / L_eff;
di_c = ( v(3) - R*i_c - lambda * f(3) * wm ) / L_eff;

% Mechanic equations
T_elec = lambda*( f(1)*i_a + f(2)*i_b + f(3)*i_c ); % torque eléctrico
dwm = ( T_elec - b*wm - Tl ) / J;


% Electric angle
dtheta = (P/2) * wm;

dX = [di_a; di_b; di_c; dwm; dtheta];

end

== matlab function LongLatDriveline/LateralController/HOSMC_IntegralBlocksSuperTwisting/MATLAB Function2 ==
  data: u input; y output
function y = fcn(u)
L = pi;
e = 25;

y = L.*tanh(u./e);

== matlab function LongLatDriveline/LateralController/SMC_Conventional1 ==
  data: U output size=1; E input; Vx input; C_af parameter; g parameter; C_ar parameter; lf parameter; lr parameter; Iz parameter; m parameter
% ******************* Lateral dynamic controller *********************
%*********************************************************************
% Author: L.Arturo Torres-Romero
% Date: 22-10-2020
% This controller controlls the direction of a car, based in the dynamics
% described  in the next link and using the conventional sliding mode control 
% formulation with the procedure of converting to regular form: 
% https://www.researchgate.net/publication/340166902_LATERAL_VEHICLE_DYNAMICS_AND_CONTROLLERS_DESIGN
%******************* PARAMETERS DESCRIPTIONS **********************
%******************************************************************
% m: vehicle mass
% g: gravity
% C_af : Cornering  stiffness  of  front  wheels.
% C_ar : Cornering  stiffness  of  rear  wheels.
% lf : distance fron the center of gravity to the front wheel axis.
% lr : distance fron the center of gravity to the rear wheel axis.
% Iz : this is the momentum of inertia of the vehicle respect the z axis.
%******************************************************************
%******************* INPUTS DESCRIPTIONS **************************
%******************************************************************
% E:   (column vector)[e1;de1;e2;de2] states of the state space of 
%       the system that includes the errors as follows:
%      e1  : is the lateral position error respect the road.
%      de1 : derivative of e1.
%      e2  : is the yaw angle error with respect the road. 
%      de2 : derivarive of the e2.
% Vx: Logitudinal velocity.

%******************************************************************
% ******************* OUTPUTS DESCRIPTIONS ************************
%******************************************************************
% U: control coutput in radians. Angle of the frontal wheels respect to the
%    longitudinal axis
% isCtrl: when true means that the matrix Mc has full rank, and hence, the
%         system is controllable
%******************************************************************

function U = SMC_ConventionalCtrl(E, Vx, C_af, g, C_ar, lf, lr, Iz, m) % pd polos deseados
X = [0; 0; 0; 0];
X(1) = E(1);
X(2) = E(2);
X(3) = E(3);
X(4) = E(4);
n = 16;
lambda_1 = -1;
lambda_2 = -2;
%**************************************************
%******* Matrix A formulation *********************
A22 = -(2*C_af + 2*C_ar)/(m*Vx);
A23 = (2*C_af + 2*C_ar)/m;
A24 = (-2*C_af*lf + 2*C_ar*lr)/(m*Vx);
A42 = -(2*C_af*lf - 2*C_ar*lr)/(Iz*Vx);
A43 = (2*C_af*lf - 2*C_ar*lr)/Iz;
A44 = -(2*C_af*lf^2 + 2*C_ar*lr^2)/(Iz*Vx);

A = [0 1 0 0;0 A22 A23 A24;0 0 0 1;0 A42 A43 A44];
%**************************************************

%**************************************************
%******* Matrix B1 formulation ********************
B1_2 = 2*C_af/m;
B1_4 = 2*C_af*lf/Iz;

B1 = [0;B1_2;0;B1_4];
%***************************************************

%***************************************************
%******* Matrix B2 formulation *********************
B2_2 = -(2*C_af*lf - 2*C_ar*lr)/(m*Vx) - Vx;
B2_4 = -(2*C_af*lf^2 + 2*C_ar*lr^2)/(Iz*Vx);

B2 = [0;B2_2;0;B2_4];
%***************************************************


%***************************************************
%******* Matrix B3 formulation *********************
B3 = [0;g;0;0];
%***************************************************
x1 = X(1);
x2 = X(2);
x3 = X(3);
x4 = X(4);

%%%%%% this is with S2 = inv(B_2)
% sigma1 = -(lambda_2*x1 - x2 + lambda_2*x3)/B1_2;
% sigma2 = -(lambda_1*x1 - x4 + lambda_1*x3)/B1_4;
% u1 = -(A22*x2 + A23*x3 + A24*x4 - lambda_2*x2 - lambda_2*x4 + B1_2*n*sign(sigma1))/B1_2;
% u2 = -(A42*x2 + A43*x3 + A44*x4 - lambda_1*x2 - lambda_1*x4 + B1_4*n*sign(sigma2))/B1_4;


%%%%%% this is with S2 = eye(2)
sigma1 = -(abs(B1_4)*(lambda_1*x1 - x4 + lambda_1*x3))/B1_4;
sigma2 = -(abs(B1_2)*(lambda_2*x1 - x2 + lambda_2*x3))/B1_2;
u1 = -(A42*x2 + A43*x3 + A44*x4 - lambda_1*x2 - lambda_1*x4 + n*sign(B1_4)*sign(sigma1))/B1_4;
u2 = -(A22*x2 + A23*x3 + A24*x4 - lambda_2*x2 - lambda_2*x4 + n*sign(B1_2)*sign(sigma2))/B1_2;

ctrlVal =  (u2+u1)/2;

U = real(ctrlVal);    



%*****************************************************************************
%******* Live script for help in calculus of the controller ************
% 
% format rational
% syms A B Q R Tr B1_2 B1_4 A22 A23 A24 A42 A43 A44
% A = [0 1 0 0;0 A22 A23 A24;0 0 0 1;0 A42 A43 A44]
% B = [0 0;B1_2 0;0 0;0 B1_4]
% 
% [Q R] = qr(sym(B))
% 
% Tr= flipud(Q') % we need the cero part in the superior part
% rank(Tr)
% 
% B_ = Tr*B
% 
% A_ = Tr*A*inv(Tr)
% 
% % A_ matrix partition
% A_11 = A_(1:2,1:2)
% A_12 = A_(1:2,3:4)
% A_21 = A_(3:4,1:2)
% A_22 = A_(3:4,3:4)
% 
% syms M M11 M12 M21 M22 lambda_1 lambda_2
% M = [M11 M12;M21 M22];
% eqeigen = [lambda_1;lambda_2] == A_11 - A_12*M;
% H = solve(eqeigen,M);
% M_ = [H.M11 H.M12;H.M21 H.M22]
% 
% S2 = eye(2);
% %S2 = inv(B_(3:4,:))
% S = S2*[M_ eye(2)]*Tr;
% disp("surface S: ")
% expand(S)
% 
% syms n sigma_ x1 x2 x3 x4 u1 u2
% X = [x1;x2;x3;x4];
% U = [u1;u2];
% 
% SIGMA = S*X;
% Sigma_1 = simplify(SIGMA(1))
% Sigma_2 = simplify(SIGMA(2))
% 
% eqsolution = -n*sign(sigma_) == S*(A*X + B*U)
% sol1 = solve(eqsolution(1),u2);
% sol2 = solve(eqsolution(2),u1);
% 
% simplify(sol1)
% simplify(sol2)

== matlab function LongLatDriveline/Tyre ModelV1/MagicFormula ==
  data: X input; Y output; F_zf input
%BASED ON
%Massimo Guiggiani, The Science of Vehicle Dynamics, Pisa, Italy, Springer Netherlands, 2014.
%Chapter 2.12
%The values of the MF were obtained from the graph in fig. 2.22
function Y = XTireForce(X, F_zf) 
% B stiffness factor
% C shape factor
% D peak value
% E curvature factor
% Sh horizontal shift
% Sv vertical shift

Sh = 0;% Sh horizontal shift
Sv = 0; %vertical shift

D = 3; % ym, maximum value Experimental from graph
C = 1.5;
B = 20;
E = 0;

x = X-Sh;
gamma = C*atan(B*x-E*(B*x-atan(B*x)));
y = F_zf*D*sin(gamma);
Y = (y - Sv);

== matlab function LongLatDriveline/SteerActuator/BLDCWRack/BLDC_AngleCtrl2/Back EMF ==
  data: X input; Fabc output
function Fabc = fcn(X)
Fabc = [0;0;0];
    theta = mod(X(5),2*pi); %X(4)
    %theta = mod(X,2*pi);
    
    if (0<=theta)&&(theta<(pi/6))
        Fa = (6/pi)*theta;
    elseif ((pi/6)<=theta)&&(theta<(5*pi/6))
        Fa = 1;
    elseif ((5*pi/6<=theta))&&(theta<(7*pi/6))
        Fa = (6/pi)*(pi-theta);
    elseif ((7*pi/6)<=theta)&&(theta<(11*pi/6))
        Fa = -1;
    elseif ((11*pi/6)<=theta)&&(theta<(2*pi))
        Fa = (6/pi)*(theta-2*pi);
    else
        Fa = NaN;
    end
    
    if (0<=theta)&&(theta<(3*pi/6))
        Fb = -1;
    elseif ((3*pi/6)<=theta)&&(theta<(5*pi/6))
        Fb = (6/pi)*(theta-(2*pi)/3);
    elseif ((5*pi/6)<=theta)&&(theta<(9*pi/6))
        Fb = 1;
    elseif ((9*pi/6)<=theta)&&(theta<(11*pi/6))
        Fb = (6/pi)*(-theta+(5*pi)/3);
    elseif ((11*pi/6)<=theta)&&(theta<(2*pi))
        Fb = -1;
    else
        Fb = NaN;
    end
    
    if (0<=theta)&&(theta<(pi/6))
        Fc = 1;
    elseif ((pi/6)<=theta)&&(theta<(3*pi/6))
        Fc = (6/pi)*(pi/3-theta);
    elseif ((3*pi/6)<=theta)&&(theta<(7*pi/6))
        Fc = -1;
    elseif ((7*pi/6)<=theta)&&(theta<(9*pi/6))
        Fc = (6/pi)*(theta-(4*pi)/3);
    elseif ((9*pi/6)<=theta)&&(theta<(2*pi))
        Fc = 1;
    else
        Fc = NaN; 
    end
    
    
%     
     %Fa = sin(theta);
     %Fb = sin(theta - 2*pi/3);
     %Fc = sin(theta + 2*pi/3);
    
    Fabc = [Fa;Fb;Fc];
end

== matlab function LongLatDriveline/SteerActuator/BLDCWRack/BLDC_AngleCtrl2/InvParkClarke ==
  data: X_dq input; Y_abc output; theta input
function Y_abc = fcn(X_dq, theta)
Y_abc = [0;0;0];
X_dq0 = [X_dq; 0];

%inverse Park-Clarke power invariant
iT_PC = sqrt(2/3)*[cos(theta)          -sin(theta)            1/sqrt(2); ...
                  cos(theta-2*pi/3)   -sin(theta-2*pi/3)     1/sqrt(2); ...
                  cos(theta+2*pi/3)   -sin(theta+2*pi/3)     1/sqrt(2)];
%               
              
 %inverse Park-Clarke amplitude invariant
% iT_PC = [cos(theta)          -sin(theta)            1; ...
%          cos(theta-2*pi/3)   -sin(theta-2*pi/3)     1; ...
%          cos(theta+2*pi/3)   -sin(theta+2*pi/3)     1];



Y_abc =iT_PC*X_dq0;
end

== matlab function LongLatDriveline/SteerActuator/BLDCWRack/BLDC_AngleCtrl2/ParkClarke ==
  data: X_abc input; Y_dq output; theta input
function Y_dq = fcn(X_abc, theta)
Y_dq = [0;0];
% Park clarke transform eliminating the third element
PC_T = (sqrt(2)/2)*[sqrt(3)*cos(theta)  sin(theta)  -sin(theta) ; ...
                    -sqrt(3)*sin(theta)  cos(theta)  -cos(theta)];

Y_dq =PC_T*X_abc;
end

== matlab function LongLatDriveline/SteerActuator/BLDCWRack/RackSubsystem/SteerMechanics ==
  data: dd input; dWs input; Ws input; Vx input; Ts output; m parameter; g parameter; t_f output; t_a output
function [Ts,t_f,t_a] = fcn(dd, dWs, Ws,Vx, m, g)

Fz = (m*g)/2; % N.  4 tires
J_s = 0.024; %kg
B_s = 0.00172; % Nm*s/deg
epsilon = 0.1;
Nl = 0.00006;


t_f = -Fz * tanh(Ws/(epsilon)); % derivative of dd is equivalent 
    % to 1/Nm of the electrical angular speed
t_a = -Fz*Vx*sin(dd);


Ts = Nl*(J_s*dWs + B_s*Ws - t_a - t_f);

== matlab function LongLatDriveline/SteerActuator/BLDC_AngleCtrl/BLDC abc model ==
  data: X input; f input; v input; dX output; Tl input; R parameter; L parameter; M parameter; J parameter; b parameter; P parameter; lambda parameter
function dX = fcn(X,f,v,Tl, R, L, M, J, b, P, lambda)
% X = [i_a; i_b; i_c; wm; theta_elec]
% f = [f1; f2; f3]  (0..1)
% v = [v1; v2; v3]  (example v = 12.*f)
% Tl = scalar torque load)
% lambda = ke = kt (V·s/rad = N·m/A)
% P = poles qty (pole pairs = P/2
%
% delivers dX = [di_a; di_b; di_c; dwm; dtheta_elec]

% sanity checks
if numel(f)~=3 || numel(v)~=3
    error('f and v must be vectors 3x1.');
end

% effective electric parameters
L_eff = L - M;
if L_eff <= 0
    error('L - M must be possitive. Check M.');
end


% states
i_a = X(1); i_b = X(2); i_c = X(3);
wm  = X(4); theta = X(5);


% electric equations (phase to phase)
di_a = ( v(1) - R*i_a - lambda * f(1) * wm ) / L_eff;
di_b = ( v(2) - R*i_b - lambda * f(2) * wm ) / L_eff;
di_c = ( v(3) - R*i_c - lambda * f(3) * wm ) / L_eff;

% Mechanic equations
T_elec = lambda*( f(1)*i_a + f(2)*i_b + f(3)*i_c ); % torque eléctrico
dwm = ( T_elec - b*wm - Tl ) / J;


% Electric angle
dtheta = (P/2) * wm;

dX = [di_a; di_b; di_c; dwm; dtheta];

end
